simulink model "INV_ASPICE_Inverter_Demo"  (R2026a)
settings: Solver=FixedStepDiscrete  StopTime=0.28  FixedStep=1e-05
InitFcn:
  | run(fullfile(fileparts(get_param(bdroot,'FileName')),'init_INV_ASPICE_demo.m'))
values from neighbouring files (symbols this model uses):
  INV_ElectricalFreq = 50.0    (= 50)    [init_INV_ASPICE_demo.m]
  INV_LoadL = 2.5e-3    (= 0.0025)    [init_INV_ASPICE_demo.m]
  INV_LoadR = 0.50    (= 0.5)    [init_INV_ASPICE_demo.m]
  INV_LongOvEnd = 0.230    (= 0.23)    [init_INV_ASPICE_demo.m]
  INV_LongOvStart = 0.100    (= 0.1)    [init_INV_ASPICE_demo.m]
  INV_ModulationIndex = 0.80    (= 0.8)    [init_INV_ASPICE_demo.m]
  INV_OV_DebounceCount = round(INV_OV_DebounceTime / INV_Ts)    [init_INV_ASPICE_demo.m]
  INV_OV_ResetThreshold = 400.0    (= 400)    [init_INV_ASPICE_demo.m]
  INV_OV_SetThreshold = 420.0    (= 420)    [init_INV_ASPICE_demo.m]
  INV_ResetPulseWidth = 0.001    [init_INV_ASPICE_demo.m]
  INV_ResetTime = 0.250    (= 0.25)    [init_INV_ASPICE_demo.m]
  INV_ShortOvEnd = 0.080    (= 0.08)    [init_INV_ASPICE_demo.m]
  INV_ShortOvStart = 0.030    (= 0.03)    [init_INV_ASPICE_demo.m]
  INV_Tpwm = 1.0 / INV_PwmFrequency    (= 0.0001)    [init_INV_ASPICE_demo.m]
  INV_Ts = 1.0e-5    (= 1e-05)    [init_INV_ASPICE_demo.m]
  INV_VdcNom = 400.0    (= 400)    [init_INV_ASPICE_demo.m]
libraries: simulink x1
settings Model: Creator=smart  LastModifiedBy=smart

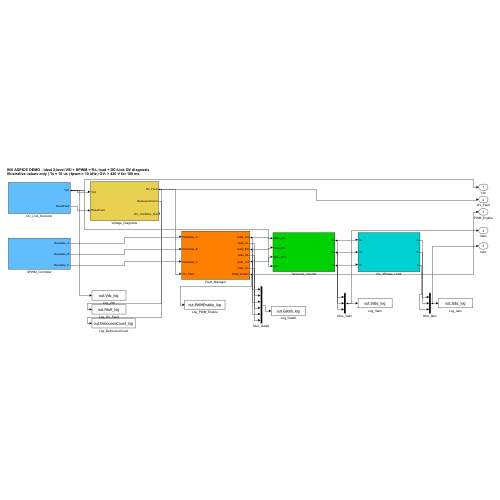
[thumbnail: Simulink's stored preview of the top-level diagram]
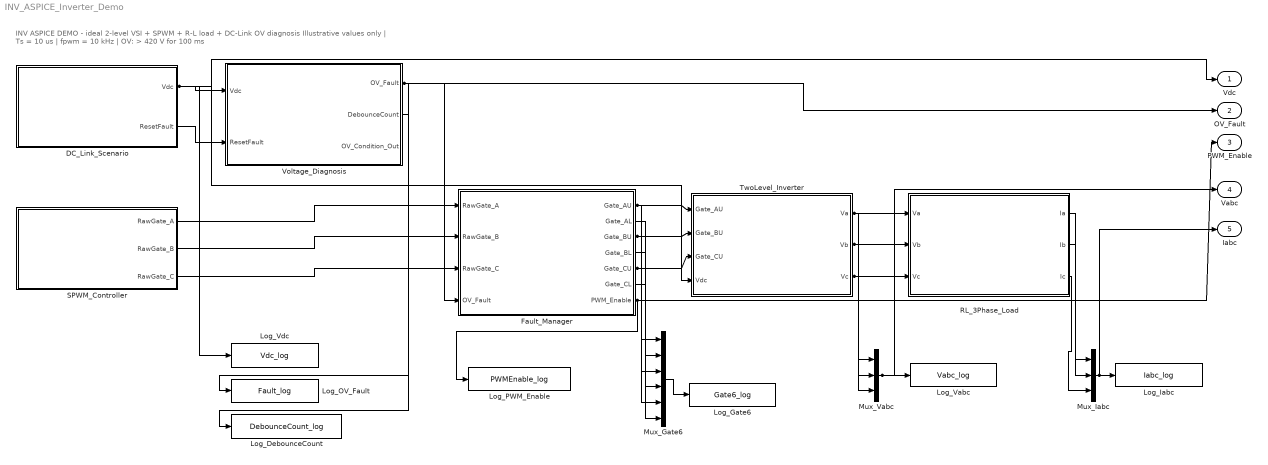
== system INV_ASPICE_Inverter_Demo ==
  note: INV ASPICE DEMO - ideal 2-level VSI + SPWM + R-L load + DC-Link OV diagnosis
      | Illustrative values only | Ts = 10 us | fpwm = 10 kHz | OV: > 420 V for 100 ms
  DC_Link_Scenario : Subsystem
  Fault_Manager : Subsystem
  Log_DebounceCount : ToWorkspace  VariableName=DebounceCount_log  SaveFormat=Timeseries  SampleTime=-1
      settings: MaxDataPoints=1e6
  Log_Gate6 : ToWorkspace  VariableName=Gate6_log  SaveFormat=Timeseries  SampleTime=-1
      settings: MaxDataPoints=1e6
  Log_Iabc : ToWorkspace  VariableName=Iabc_log  SaveFormat=Timeseries  SampleTime=-1
      settings: MaxDataPoints=1e6
  Log_OV_Fault : ToWorkspace  VariableName=Fault_log  SaveFormat=Timeseries  SampleTime=-1
      settings: MaxDataPoints=1e6
  Log_PWM_Enable : ToWorkspace  VariableName=PWMEnable_log  SaveFormat=Timeseries  SampleTime=-1
      settings: MaxDataPoints=1e6
  Log_Vabc : ToWorkspace  VariableName=Vabc_log  SaveFormat=Timeseries  SampleTime=-1
      settings: MaxDataPoints=1e6
  Log_Vdc : ToWorkspace  VariableName=Vdc_log  SaveFormat=Timeseries  SampleTime=-1
      settings: MaxDataPoints=1e6
  Mux_Gate6 : Mux  Inputs=6
  Mux_Iabc : Mux  Inputs=3
  Mux_Vabc : Mux  Inputs=3
  RL_3Phase_Load : Subsystem
  SPWM_Controller : Subsystem
  TwoLevel_Inverter : Subsystem
  Voltage_Diagnosis : Subsystem
  Vdc : Outport
  OV_Fault : Outport  Port=2
  PWM_Enable : Outport  Port=3
  Vabc : Outport  Port=4
  Iabc : Outport  Port=5
  wires:
  DC_Link_Scenario/1(Vdc) -> Voltage_Diagnosis/1(Vdc), TwoLevel_Inverter/4(Vdc), Log_Vdc/1, Vdc/1
  DC_Link_Scenario/2(ResetFault) -> Voltage_Diagnosis/2(ResetFault)
  SPWM_Controller/1(RawGate_A) -> Fault_Manager/1(RawGate_A)
  SPWM_Controller/2(RawGate_B) -> Fault_Manager/2(RawGate_B)
  SPWM_Controller/3(RawGate_C) -> Fault_Manager/3(RawGate_C)
  Voltage_Diagnosis/1(OV_Fault) -> Fault_Manager/4(OV_Fault), Log_OV_Fault/1, OV_Fault/1
  Fault_Manager/1(Gate_AU) -> TwoLevel_Inverter/1(Gate_AU), Mux_Gate6/1
  Fault_Manager/3(Gate_BU) -> TwoLevel_Inverter/2(Gate_BU), Mux_Gate6/3
  Fault_Manager/5(Gate_CU) -> TwoLevel_Inverter/3(Gate_CU), Mux_Gate6/5
  TwoLevel_Inverter/1(Va) -> RL_3Phase_Load/1(Va), Mux_Vabc/1
  TwoLevel_Inverter/2(Vb) -> RL_3Phase_Load/2(Vb), Mux_Vabc/2
  TwoLevel_Inverter/3(Vc) -> RL_3Phase_Load/3(Vc), Mux_Vabc/3
  RL_3Phase_Load/1(Ia) -> Mux_Iabc/1
  RL_3Phase_Load/2(Ib) -> Mux_Iabc/2
  RL_3Phase_Load/3(Ic) -> Mux_Iabc/3
  Fault_Manager/2(Gate_AL) -> Mux_Gate6/2
  Fault_Manager/4(Gate_BL) -> Mux_Gate6/4
  Fault_Manager/6(Gate_CL) -> Mux_Gate6/6
  Fault_Manager/7(PWM_Enable) -> Log_PWM_Enable/1, PWM_Enable/1
  Voltage_Diagnosis/2(DebounceCount) -> Log_DebounceCount/1
  Mux_Gate6/1 -> Log_Gate6/1
  Mux_Vabc/1 -> Log_Vabc/1, Vabc/1
  Mux_Iabc/1 -> Log_Iabc/1, Iabc/1

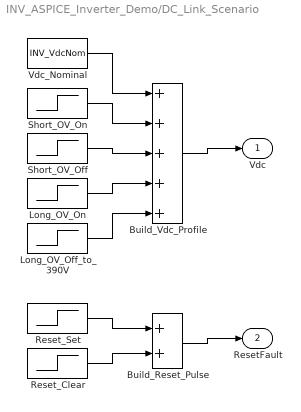
== system INV_ASPICE_Inverter_Demo/DC_Link_Scenario ==
  Build_Reset_Pulse : Sum
  Build_Vdc_Profile : Sum  Inputs=+++++
  Long_OV_Off_to_390V : Step  Time=INV_LongOvEnd  FinalValue=-40  SampleTime=INV_Ts
  Long_OV_On : Step  Time=INV_LongOvStart  FinalValue=30  SampleTime=INV_Ts
  Reset_Clear : Step  Time=INV_ResetTime + INV_ResetPulseWidth  FinalValue=-1  SampleTime=INV_Ts
  Reset_Set : Step  Time=INV_ResetTime  SampleTime=INV_Ts
  Short_OV_Off : Step  Time=INV_ShortOvEnd  FinalValue=-30  SampleTime=INV_Ts
  Short_OV_On : Step  Time=INV_ShortOvStart  FinalValue=30  SampleTime=INV_Ts
  Vdc_Nominal : Constant  Value=INV_VdcNom
  Vdc : Outport
  ResetFault : Outport  Port=2
  wires:
  Vdc_Nominal/1 -> Build_Vdc_Profile/1
  Short_OV_On/1 -> Build_Vdc_Profile/2
  Short_OV_Off/1 -> Build_Vdc_Profile/3
  Long_OV_On/1 -> Build_Vdc_Profile/4
  Long_OV_Off_to_390V/1 -> Build_Vdc_Profile/5
  Build_Vdc_Profile/1 -> Vdc/1
  Reset_Set/1 -> Build_Reset_Pulse/1
  Reset_Clear/1 -> Build_Reset_Pulse/2
  Build_Reset_Pulse/1 -> ResetFault/1

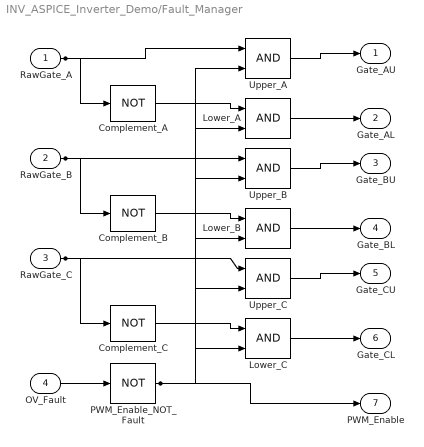
== system INV_ASPICE_Inverter_Demo/Fault_Manager ==
  RawGate_A : Inport
  RawGate_B : Inport  Port=2
  RawGate_C : Inport  Port=3
  OV_Fault : Inport  Port=4
  Complement_A : Logic  Operator=NOT  AllPortsSameDT=off  OutDataTypeStr=boolean
  Complement_B : Logic  Operator=NOT  AllPortsSameDT=off  OutDataTypeStr=boolean
  Complement_C : Logic  Operator=NOT  AllPortsSameDT=off  OutDataTypeStr=boolean
  Lower_A : Logic  AllPortsSameDT=off  OutDataTypeStr=boolean
  Lower_B : Logic  AllPortsSameDT=off  OutDataTypeStr=boolean
  Lower_C : Logic  AllPortsSameDT=off  OutDataTypeStr=boolean
  PWM_Enable_NOT_Fault : Logic  Operator=NOT  AllPortsSameDT=off  OutDataTypeStr=boolean
  Upper_A : Logic  AllPortsSameDT=off  OutDataTypeStr=boolean
  Upper_B : Logic  AllPortsSameDT=off  OutDataTypeStr=boolean
  Upper_C : Logic  AllPortsSameDT=off  OutDataTypeStr=boolean
  Gate_AU : Outport
  Gate_AL : Outport  Port=2
  Gate_BU : Outport  Port=3
  Gate_BL : Outport  Port=4
  Gate_CU : Outport  Port=5
  Gate_CL : Outport  Port=6
  PWM_Enable : Outport  Port=7
  wires:
  OV_Fault/1 -> PWM_Enable_NOT_Fault/1
  RawGate_A/1 -> Upper_A/1, Complement_A/1
  PWM_Enable_NOT_Fault/1 -> Upper_A/2, Lower_A/2, Upper_B/2, Lower_B/2, Upper_C/2, Lower_C/2, PWM_Enable/1
  Complement_A/1 -> Lower_A/1
  Upper_A/1 -> Gate_AU/1
  Lower_A/1 -> Gate_AL/1
  RawGate_B/1 -> Upper_B/1, Complement_B/1
  Complement_B/1 -> Lower_B/1
  Upper_B/1 -> Gate_BU/1
  Lower_B/1 -> Gate_BL/1
  RawGate_C/1 -> Upper_C/1, Complement_C/1
  Complement_C/1 -> Lower_C/1
  Upper_C/1 -> Gate_CU/1
  Lower_C/1 -> Gate_CL/1

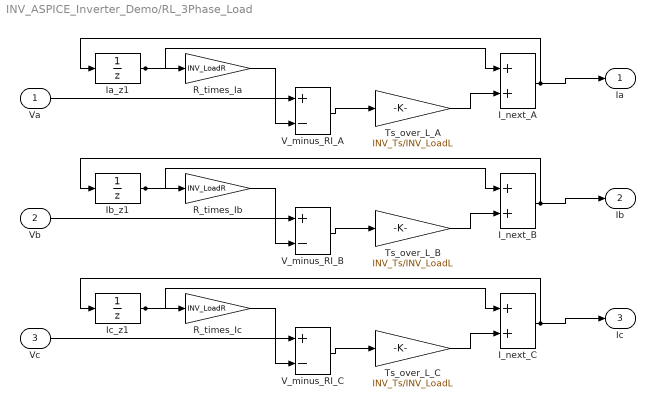
== system INV_ASPICE_Inverter_Demo/RL_3Phase_Load ==
  Va : Inport
  Vb : Inport  Port=2
  Vc : Inport  Port=3
  I_next_A : Sum
  I_next_B : Sum
  I_next_C : Sum
  Ia_z1 : UnitDelay  SampleTime=INV_Ts
  Ib_z1 : UnitDelay  SampleTime=INV_Ts
  Ic_z1 : UnitDelay  SampleTime=INV_Ts
  R_times_Ia : Gain  Gain=INV_LoadR
  R_times_Ib : Gain  Gain=INV_LoadR
  R_times_Ic : Gain  Gain=INV_LoadR
  Ts_over_L_A : Gain  Gain=INV_Ts/INV_LoadL
  Ts_over_L_B : Gain  Gain=INV_Ts/INV_LoadL
  Ts_over_L_C : Gain  Gain=INV_Ts/INV_LoadL
  V_minus_RI_A : Sum  Inputs=+-
  V_minus_RI_B : Sum  Inputs=+-
  V_minus_RI_C : Sum  Inputs=+-
  Ia : Outport
  Ib : Outport  Port=2
  Ic : Outport  Port=3
  wires:
  Ia_z1/1 -> R_times_Ia/1, I_next_A/1
  Va/1 -> V_minus_RI_A/1
  R_times_Ia/1 -> V_minus_RI_A/2
  V_minus_RI_A/1 -> Ts_over_L_A/1
  Ts_over_L_A/1 -> I_next_A/2
  I_next_A/1 -> Ia_z1/1, Ia/1
  Ib_z1/1 -> R_times_Ib/1, I_next_B/1
  Vb/1 -> V_minus_RI_B/1
  R_times_Ib/1 -> V_minus_RI_B/2
  V_minus_RI_B/1 -> Ts_over_L_B/1
  Ts_over_L_B/1 -> I_next_B/2
  I_next_B/1 -> Ib_z1/1, Ib/1
  Ic_z1/1 -> R_times_Ic/1, I_next_C/1
  Vc/1 -> V_minus_RI_C/1
  R_times_Ic/1 -> V_minus_RI_C/2
  V_minus_RI_C/1 -> Ts_over_L_C/1
  Ts_over_L_C/1 -> I_next_C/2
  I_next_C/1 -> Ic_z1/1, Ic/1

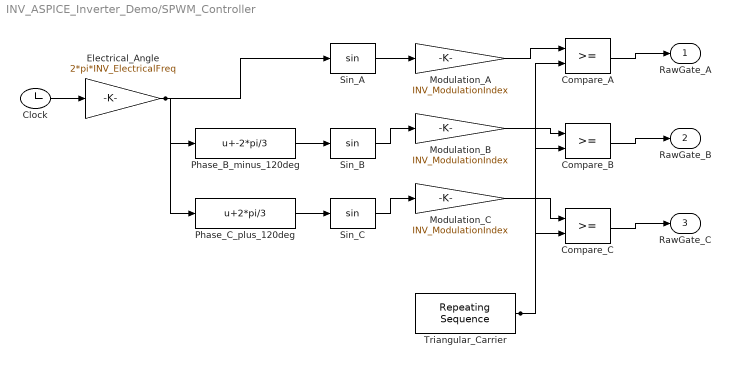
== system INV_ASPICE_Inverter_Demo/SPWM_Controller ==
  Clock : Clock
  Compare_A : RelationalOperator  OutDataTypeStr=boolean  RndMeth=Simplest  InputSameDT=off
  Compare_B : RelationalOperator  OutDataTypeStr=boolean  RndMeth=Simplest  InputSameDT=off
  Compare_C : RelationalOperator  OutDataTypeStr=boolean  RndMeth=Simplest  InputSameDT=off
  Electrical_Angle : Gain  Gain=2*pi*INV_ElectricalFreq
  Modulation_A : Gain  Gain=INV_ModulationIndex
  Modulation_B : Gain  Gain=INV_ModulationIndex
  Modulation_C : Gain  Gain=INV_ModulationIndex
  Phase_B_minus_120deg : Bias  Bias=-2*pi/3  SaturateOnIntegerOverflow=off
  Phase_C_plus_120deg : Bias  Bias=2*pi/3  SaturateOnIntegerOverflow=off
  Sin_A : Trigonometry
  Sin_B : Trigonometry
  Sin_C : Trigonometry
  Triangular_Carrier : simulink/Sources/Repeating Sequence  rep_seq_t=[0 INV_Tpwm/2 INV_Tpwm]  rep_seq_y=[-1 1 -1]
  RawGate_A : Outport
  RawGate_B : Outport  Port=2
  RawGate_C : Outport  Port=3
  wires:
  Modulation_A/1 -> Compare_A/1
  Triangular_Carrier/1 -> Compare_A/2, Compare_B/2, Compare_C/2
  Compare_A/1 -> RawGate_A/1
  Modulation_B/1 -> Compare_B/1
  Compare_B/1 -> RawGate_B/1
  Modulation_C/1 -> Compare_C/1
  Compare_C/1 -> RawGate_C/1
  Clock/1 -> Electrical_Angle/1
  Electrical_Angle/1 -> Sin_A/1, Phase_B_minus_120deg/1, Phase_C_plus_120deg/1
  Phase_B_minus_120deg/1 -> Sin_B/1
  Phase_C_plus_120deg/1 -> Sin_C/1
  Sin_A/1 -> Modulation_A/1
  Sin_B/1 -> Modulation_B/1
  Sin_C/1 -> Modulation_C/1

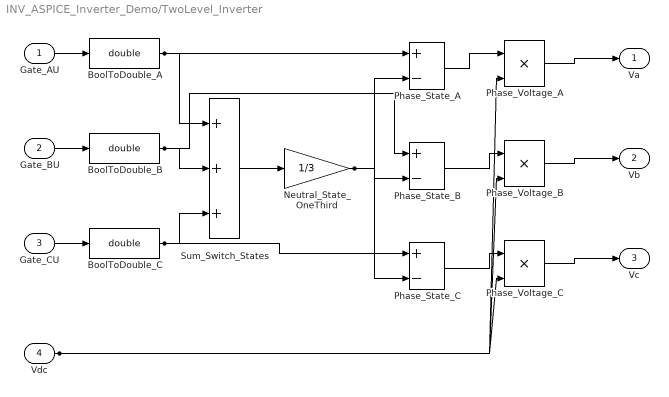
== system INV_ASPICE_Inverter_Demo/TwoLevel_Inverter ==
  Gate_AU : Inport
  Gate_BU : Inport  Port=2
  Gate_CU : Inport  Port=3
  Vdc : Inport  Port=4
  BoolToDouble_A : DataTypeConversion  OutDataTypeStr=double  SaturateOnIntegerOverflow=off  RndMeth=Floor
  BoolToDouble_B : DataTypeConversion  OutDataTypeStr=double  SaturateOnIntegerOverflow=off  RndMeth=Floor
  BoolToDouble_C : DataTypeConversion  OutDataTypeStr=double  SaturateOnIntegerOverflow=off  RndMeth=Floor
  Neutral_State_OneThird : Gain  Gain=1/3
  Phase_State_A : Sum  Inputs=+-
  Phase_State_B : Sum  Inputs=+-
  Phase_State_C : Sum  Inputs=+-
  Phase_Voltage_A : Product  Inputs=**
  Phase_Voltage_B : Product  Inputs=**
  Phase_Voltage_C : Product  Inputs=**
  Sum_Switch_States : Sum  Inputs=+++
  Va : Outport
  Vb : Outport  Port=2
  Vc : Outport  Port=3
  wires:
  Gate_AU/1 -> BoolToDouble_A/1
  Gate_BU/1 -> BoolToDouble_B/1
  Gate_CU/1 -> BoolToDouble_C/1
  BoolToDouble_A/1 -> Sum_Switch_States/1, Phase_State_A/1
  BoolToDouble_B/1 -> Sum_Switch_States/2, Phase_State_B/1
  BoolToDouble_C/1 -> Sum_Switch_States/3, Phase_State_C/1
  Sum_Switch_States/1 -> Neutral_State_OneThird/1
  Neutral_State_OneThird/1 -> Phase_State_A/2, Phase_State_B/2, Phase_State_C/2
  Phase_State_A/1 -> Phase_Voltage_A/1
  Vdc/1 -> Phase_Voltage_A/2, Phase_Voltage_B/2, Phase_Voltage_C/2
  Phase_Voltage_A/1 -> Va/1
  Phase_State_B/1 -> Phase_Voltage_B/1
  Phase_Voltage_B/1 -> Vb/1
  Phase_State_C/1 -> Phase_Voltage_C/1
  Phase_Voltage_C/1 -> Vc/1

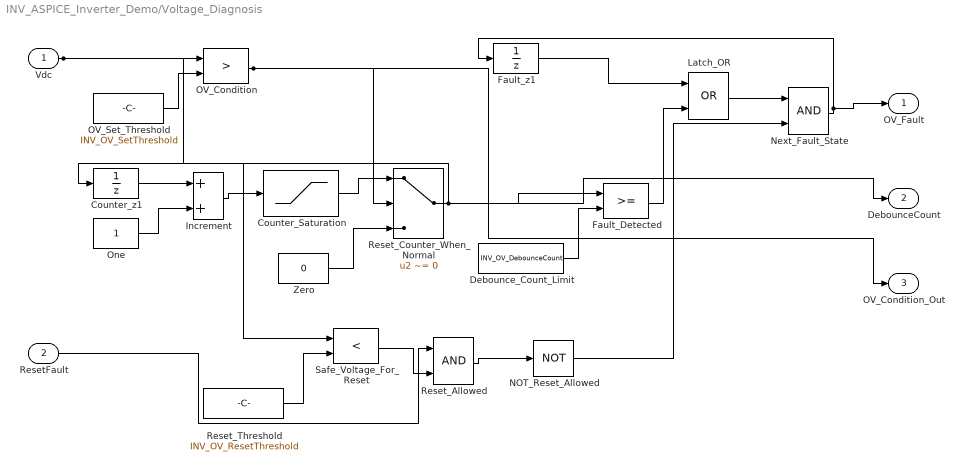
== system INV_ASPICE_Inverter_Demo/Voltage_Diagnosis ==
  Vdc : Inport
  ResetFault : Inport  Port=2
  Counter_Saturation : Saturate  UpperLimit=INV_OV_DebounceCount  LowerLimit=0
  Counter_z1 : UnitDelay  SampleTime=INV_Ts
  Debounce_Count_Limit : Constant  Value=INV_OV_DebounceCount
  Fault_Detected : RelationalOperator  OutDataTypeStr=boolean  RndMeth=Simplest  InputSameDT=off
  Fault_z1 : UnitDelay  InitialCondition=false  SampleTime=INV_Ts
  Increment : Sum
  Latch_OR : Logic  Operator=OR  AllPortsSameDT=off  OutDataTypeStr=boolean
  NOT_Reset_Allowed : Logic  Operator=NOT  AllPortsSameDT=off  OutDataTypeStr=boolean
  Next_Fault_State : Logic  AllPortsSameDT=off  OutDataTypeStr=boolean
  OV_Condition : RelationalOperator  Operator=>  OutDataTypeStr=boolean  RndMeth=Simplest  InputSameDT=off
  OV_Set_Threshold : Constant  Value=INV_OV_SetThreshold
  One : Constant
  Reset_Allowed : Logic  AllPortsSameDT=off  OutDataTypeStr=boolean
  Reset_Counter_When_Normal : Switch  Criteria=u2 ~= 0  Threshold=0.5  SaturateOnIntegerOverflow=off  InputSameDT=off
  Reset_Threshold : Constant  Value=INV_OV_ResetThreshold
  Safe_Voltage_For_Reset : RelationalOperator  Operator=<  OutDataTypeStr=boolean  RndMeth=Simplest  InputSameDT=off
  Zero : Constant  Value=0
  OV_Fault : Outport
  DebounceCount : Outport  Port=2
  OV_Condition_Out : Outport  Port=3
  wires:
  Vdc/1 -> OV_Condition/1, Safe_Voltage_For_Reset/1
  OV_Set_Threshold/1 -> OV_Condition/2
  Counter_z1/1 -> Increment/1
  One/1 -> Increment/2
  Increment/1 -> Counter_Saturation/1
  Counter_Saturation/1 -> Reset_Counter_When_Normal/1
  OV_Condition/1 -> Reset_Counter_When_Normal/2, OV_Condition_Out/1
  Zero/1 -> Reset_Counter_When_Normal/3
  Reset_Counter_When_Normal/1 -> Counter_z1/1, Fault_Detected/1, DebounceCount/1
  Debounce_Count_Limit/1 -> Fault_Detected/2
  Fault_z1/1 -> Latch_OR/1
  Fault_Detected/1 -> Latch_OR/2
  Reset_Threshold/1 -> Safe_Voltage_For_Reset/2
  ResetFault/1 -> Reset_Allowed/1
  Safe_Voltage_For_Reset/1 -> Reset_Allowed/2
  Reset_Allowed/1 -> NOT_Reset_Allowed/1
  Latch_OR/1 -> Next_Fault_State/1
  NOT_Reset_Allowed/1 -> Next_Fault_State/2
  Next_Fault_State/1 -> Fault_z1/1, OV_Fault/1
